simulink model "Kalman_Phase_NS_Simple"  (R2019b)
settings: Solver=VariableStepAuto  StartTime=0.0  StopTime=phase_ns_model.sim_dur  FixedStep=model.Ts  RelTol=1e-6
undefined symbols (not defined in the file or in its folder): phase_ns_model
libraries: dspsrcs4 x7
settings Model: Creator=isidoraradenkovic  LastModifiedBy=isidoraradenkovic

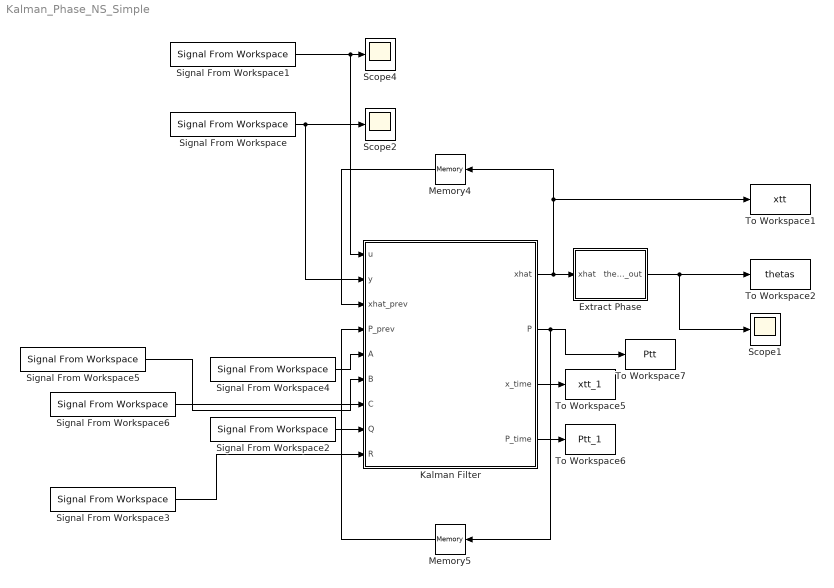
== system Kalman_Phase_NS_Simple ==
  Extract Phase : MATLAB Function  TreatAsAtomicUnit=on  SystemSampleTime=phase_ns_model.Ts
  Kalman Filter : MATLAB Function  TreatAsAtomicUnit=on
  Memory4 : Memory  InitialCondition=phase_ns_model.x_0  InheritSampleTime=on
  Memory5 : Memory  InitialCondition=phase_ns_model.P0  InheritSampleTime=on
  Scope1 : Scope
  Scope2 : Scope
  Scope4 : Scope
  Signal From Workspace : dspsrcs4/Signal From Workspace  X=input_data  Ts=phase_ns_model.Ts  nsamps=1  OutputAfterFinalValue=Cyclic repetition  ignoreOrWarnInputAndFrameLengths=off  OutputFrames=off
  Signal From Workspace1 : dspsrcs4/Signal From Workspace  X=tms_pulses  Ts=phase_ns_model.Ts  nsamps=1  OutputAfterFinalValue=Cyclic repetition  ignoreOrWarnInputAndFrameLengths=off  OutputFrames=off
  Signal From Workspace2 : dspsrcs4/Signal From Workspace  X=phase_ns_model.Q  Ts=phase_ns_model.Ts/2  nsamps=2  OutputAfterFinalValue=Cyclic repetition  ignoreOrWarnInputAndFrameLengths=off  OutputFrames=off
  Signal From Workspace3 : dspsrcs4/Signal From Workspace  X=phase_ns_model.R  Ts=phase_ns_model.Ts  nsamps=1  OutputAfterFinalValue=Cyclic repetition  ignoreOrWarnInputAndFrameLengths=off  OutputFrames=off
  Signal From Workspace4 : dspsrcs4/Signal From Workspace  X=phase_ns_model.A  Ts=phase_ns_model.Ts/2  nsamps=2  OutputAfterFinalValue=Cyclic repetition  ignoreOrWarnInputAndFrameLengths=off  OutputFrames=off
  Signal From Workspace5 : dspsrcs4/Signal From Workspace  X=phase_ns_model.B  Ts=phase_ns_model.Ts/2  nsamps=2  OutputAfterFinalValue=Cyclic repetition  ignoreOrWarnInputAndFrameLengths=off  OutputFrames=off
  Signal From Workspace6 : dspsrcs4/Signal From Workspace  X=phase_ns_model.C  Ts=phase_ns_model.Ts  nsamps=1  OutputAfterFinalValue=Cyclic repetition  ignoreOrWarnInputAndFrameLengths=off  OutputFrames=off
  To Workspace1 : ToWorkspace  VariableName=xtt  SampleTime=phase_ns_model.Ts
      settings: Save2DSignal=2-D array (concatenate along first dimension)
  To Workspace2 : ToWorkspace  VariableName=thetas  SampleTime=phase_ns_model.Ts
      settings: Save2DSignal=2-D array (concatenate along first dimension)
  To Workspace5 : ToWorkspace  VariableName=xtt_1  SampleTime=phase_ns_model.Ts
      settings: Save2DSignal=2-D array (concatenate along first dimension)
  To Workspace6 : ToWorkspace  VariableName=Ptt_1  SampleTime=phase_ns_model.Ts
      settings: Save2DSignal=2-D array (concatenate along first dimension)
  To Workspace7 : ToWorkspace  VariableName=Ptt  SampleTime=phase_ns_model.Ts
      settings: Save2DSignal=2-D array (concatenate along first dimension)
  wires:
  Kalman Filter/2(P) -> To Workspace7/1, Memory5/1
  Kalman Filter/4(P_time) -> To Workspace6/1
  Signal From Workspace6/1 -> Kalman Filter/7(C)
  Signal From Workspace/1 -> Kalman Filter/2(y), Scope2/1
  Kalman Filter/3(x_time) -> To Workspace5/1
  Signal From Workspace4/1 -> Kalman Filter/5(A)
  Signal From Workspace1/1 -> Kalman Filter/1(u), Scope4/1
  Kalman Filter/1(xhat) -> To Workspace1/1, Memory4/1, Extract Phase/1(xhat)
  Memory5/1 -> Kalman Filter/4(P_prev)
  Memory4/1 -> Kalman Filter/3(xhat_prev)
  Extract Phase/1(thetas_out) -> Scope1/1, To Workspace2/1
  Signal From Workspace2/1 -> Kalman Filter/8(Q)
  Signal From Workspace3/1 -> Kalman Filter/9(R)
  Signal From Workspace5/1 -> Kalman Filter/6(B)

== matlab function Kalman_Phase_NS_Simple/Extract Phase ==
  settings: sampleTime=model.Ts
  data: xhat input; thetas_out output
function thetas_out  = extract_phase(xhat)

thetas_out = atan2(xhat(2), xhat(1));

== matlab function Kalman_Phase_NS_Simple/Kalman Filter ==
  data: u input; xhat output; y input; xhat_prev input; P_prev input; A input; B input; C input; P output; x_time output; P_time output; Q input; R input
function [xhat, P, x_time, P_time] = phase_ns_kalman(u, y, xhat_prev, P_prev, A, B, C, Q, R)
x_time = A*xhat_prev + B*u;
P_time = A*P_prev*A'+ Q;

K = P_time*(C')*pinv(C*P_time*C' + R);
epsilon = y - C*x_time;

xhat = x_time + K*epsilon;
P = P_time - K*C*P_time;
end
